simulink model "Free_Flight_ARDrone_joystick"  (R2016b)
settings: configuration reference "AR_Drone_ConfigSet" (kept outside this file)
undefined symbols (not defined in the file): DiscIntNeverNeededParam
libraries: dspnetwork x4, simulink x4, instrumentlib x2, AR_Drone_Actuators x2, AR_Drone_Sensors x1, AR_Drone_Positioning x1, etargetslib x1
settings Model: DataDictionary=ArDroneDataDictionary.sldd  SimulationMode=external  ExtModeTrigDuration=48000  Creator=nraman  LastModifiedBy=Miguel
settings ConfigSetRef: DDName=ArDroneDataDictionary.sldd

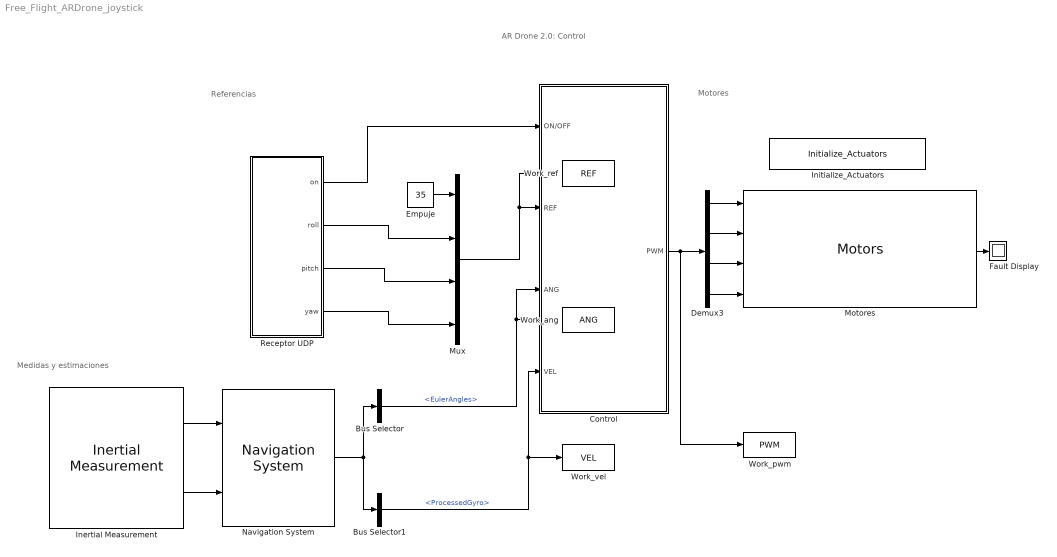
== system Free_Flight_ARDrone_joystick ==
  note: AR Drone 2.0: Control
  note: Motores
  note: Medidas y estimaciones
  note: Referencias
  Bus Selector : BusSelector  OutputSignals=EulerAngles
  Bus Selector1 : BusSelector  OutputSignals=ProcessedGyro
  Control : Subsystem
  Demux3 : Demux
  Empuje : Constant  Value=35
  Fault Display : Display
  Inertial Measurement : AR_Drone_Sensors/Inertial Measurement  Ts=1/400
  Initialize_Actuators : AR_Drone_Actuators/Initialize_Actuators  ShowSpec=on
  Motores : AR_Drone_Actuators/Motors
  Mux : Mux
  Navigation System : AR_Drone_Positioning/Navigation System
  Receptor UDP : Subsystem
  Work_ang : ToWorkspace  VariableName=ANG  SaveFormat=Structure With Time  SampleTime=0.0025
  Work_pwm : ToWorkspace  VariableName=PWM  SaveFormat=Structure With Time  SampleTime=0.0025
  Work_ref : ToWorkspace  VariableName=REF  SaveFormat=Structure With Time  SampleTime=0.0025
  Work_vel : ToWorkspace  VariableName=VEL  SaveFormat=Structure With Time  SampleTime=0.0025
  wires:
  Motores/1 -> Fault Display/1
  Demux3/1 -> Motores/1
  Demux3/2 -> Motores/2
  Demux3/3 -> Motores/3
  Demux3/4 -> Motores/4
  Inertial Measurement/1 -> Navigation System/1
  Inertial Measurement/2 -> Navigation System/2
  Navigation System/1 -> Bus Selector1/1, Bus Selector/1
  Bus Selector/1 -> Work_ang/1, Control/3(ANG)  "<EulerAngles>"
  Control/1(PWM) -> Work_pwm/1, Demux3/1
  Receptor UDP/1(on) -> Control/1(ON/OFF)
  Empuje/1 -> Mux/1
  Bus Selector1/1 -> Work_vel/1, Control/4(VEL)  "<ProcessedGyro>"
  Mux/1 -> Work_ref/1, Control/2(REF)
  Receptor UDP/2(roll) -> Mux/2
  Receptor UDP/3(pitch) -> Mux/3
  Receptor UDP/4(yaw) -> Mux/4

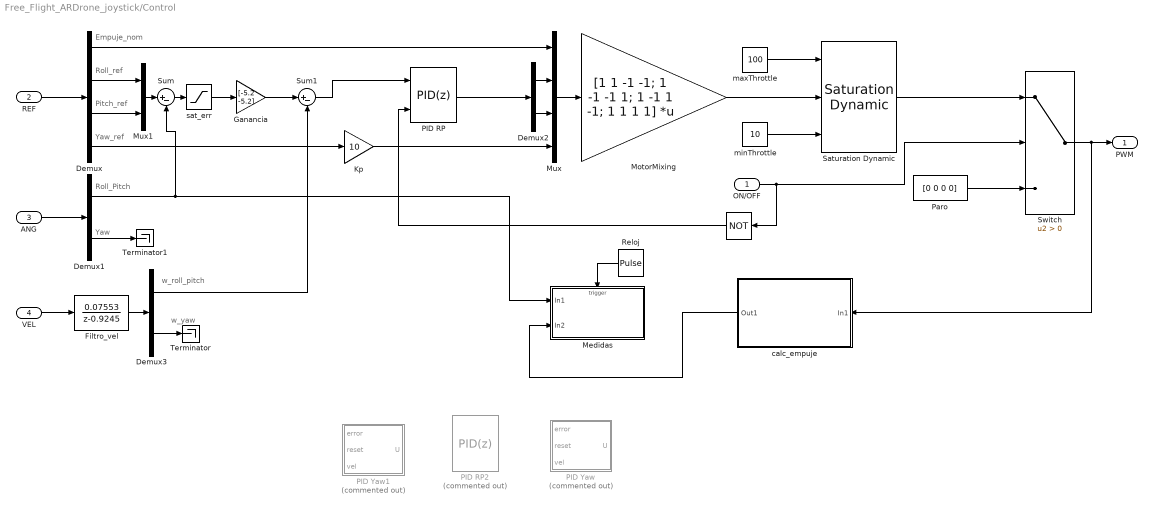
== system Free_Flight_ARDrone_joystick/Control ==
  note: Empuje_nom
  note: Roll_ref
  note: Pitch_ref
  note: Yaw_ref
  note: Roll_Pitch
  note: Yaw
  note: w_roll_pitch
  note: w_yaw
  ON/OFF : Inport
  REF : Inport  Port=2
  ANG : Inport  Port=3
  VEL : Inport  Port=4
  " " : Logic  Operator=NOT  AllPortsSameDT=off  OutDataTypeStr=boolean
  Demux : Demux
  Demux1 : Demux  Outputs=[2 1]
  Demux2 : Demux  Outputs=2
  Demux3 : Demux  Outputs=[2 1]
  Filtro_vel : DiscreteTransferFcn  Numerator=[0.07553]  Denominator=[1 -0.9245]
  Ganancia : Gain  Gain=[-5.2 -5.2]
  Kp : Gain  Gain=10
  Medidas : Subsystem
  MotorMixing : Gain  Gain=[1 1 -1 -1; 1 -1 -1 1; 1 -1 1 -1; 1 1 1 1]  Multiplication=Matrix(K*u)  ParamDataTypeStr=int16  OutDataTypeStr=int16
  Mux : Mux
  Mux1 : Mux  Inputs=2
  PID RP : simulink/Continuous/PID Controller  Controller=PID  TimeDomain=Discrete-time  SampleTime=-1  IntegratorMethod=Forward Euler  FilterMethod=Forward Euler  Form=Parallel  UseFilter=on  ControllerParametersSource=internal  P=0.5  I=0.3  D=-0.04  N=5  InitialConditionSource=internal  InitialConditionForIntegrator=0  InitialConditionForFilter=0  ExternalReset=level  LimitOutput=on  UpperSaturationLimit=30  LowerSaturationLimit=-30  LinearizeAsGain=on  AntiWindupMode=clamping  Kb=1  TrackingMode=off  Kt=1  PParamMin=[]  PParamMax=[]  IParamMin=[]  IParamMax=[]  DParamMin=[]  DParamMax=[]  NParamMin=[]  NParamMax=[]  KbParamMin=[]  KbParamMax=[]  KtParamMin=[]  KtParamMax=[]  POutMin=[]  POutMax=[]  IOutMin=[]  IOutMax=[]  DOutMin=[]  DOutMax=[]  NOutMin=[]  NOutMax=[]  KbOutMin=[]  KbOutMax=[]  KtOutMin=[]  KtOutMax=[]  IntegratorOutMin=[]  IntegratorOutMax=[]  FilterOutMin=[]  FilterOutMax=[]  SumOutMin=[]  SumOutMax=[]  SumI1OutMin=[]  SumI1OutMax=[]  SumI2OutMin=[]  SumI2OutMax=[]  SumI3OutMin=[]  SumI3OutMax=[]  SumDOutMin=[]  SumDOutMax=[]  SaturationOutMin=[]  SaturationOutMax=[]  IntegratorContinuousStateAttributes=''  IntegratorStateMustResolveToSignalObject=off  IntegratorRTWStateStorageClass=Auto  FilterContinuousStateAttributes=''  FilterStateMustResolveToSignalObject=off  FilterRTWStateStorageClass=Auto  DifferentiatorICPrevScaledInput=0  DifferentiatorOutMin=[]  DifferentiatorOutMax=[]
  PID RP2 : simulink/Continuous/PID Controller  Commented=on  Controller=PID  TimeDomain=Discrete-time  SampleTime=-1  IntegratorMethod=Forward Euler  FilterMethod=Forward Euler  Form=Parallel  UseFilter=on  ControllerParametersSource=internal  P=0.4  I=0.25  D=-0.05  N=5  InitialConditionSource=internal  InitialConditionForIntegrator=0  InitialConditionForFilter=0  ExternalReset=level  LimitOutput=on  UpperSaturationLimit=30  LowerSaturationLimit=-30  LinearizeAsGain=on  AntiWindupMode=clamping  Kb=1  TrackingMode=off  Kt=1  PParamMin=[]  PParamMax=[]  IParamMin=[]  IParamMax=[]  DParamMin=[]  DParamMax=[]  NParamMin=[]  NParamMax=[]  KbParamMin=[]  KbParamMax=[]  KtParamMin=[]  KtParamMax=[]  POutMin=[]  POutMax=[]  IOutMin=[]  IOutMax=[]  DOutMin=[]  DOutMax=[]  NOutMin=[]  NOutMax=[]  KbOutMin=[]  KbOutMax=[]  KtOutMin=[]  KtOutMax=[]  IntegratorOutMin=[]  IntegratorOutMax=[]  FilterOutMin=[]  FilterOutMax=[]  SumOutMin=[]  SumOutMax=[]  SumI1OutMin=[]  SumI1OutMax=[]  SumI2OutMin=[]  SumI2OutMax=[]  SumI3OutMin=[]  SumI3OutMax=[]  SumDOutMin=[]  SumDOutMax=[]  SaturationOutMin=[]  SaturationOutMax=[]  IntegratorContinuousStateAttributes=''  IntegratorStateMustResolveToSignalObject=off  IntegratorRTWStateStorageClass=Auto  FilterContinuousStateAttributes=''  FilterStateMustResolveToSignalObject=off  FilterRTWStateStorageClass=Auto  DifferentiatorICPrevScaledInput=0  DifferentiatorOutMin=[]  DifferentiatorOutMax=[]
  PID Yaw : Subsystem  Commented=on
  PID Yaw1 : Subsystem  Commented=on
  Paro : Constant  Value=[0 0 0 0]  OutDataTypeStr=int16
  Reloj : DiscretePulseGenerator  PulseType=Time based  Period=0.1  PulseWidth=50
  Saturation Dynamic : simulink/Discontinuities/Saturation Dynamic  OutMin=[]  OutMax=[]  OutDataTypeStr=Inherit: Same as second input  OutDataType=fixdt(1, 16)  OutScaling=2^-10  DoSatur=off
  Sum : Sum  Inputs=|+-
  Sum1 : Sum  Inputs=|+-
  Switch : Switch  Criteria=u2 > Threshold
  Terminator : Terminator
  Terminator1 : Terminator
  calc_empuje : Subsystem
  maxThrottle : Constant  Value=100  OutDataTypeStr=int16  SampleTime=-1
  minThrottle : Constant  Value=10  OutDataTypeStr=int16
  sat_err : Saturate  UpperLimit=[20 20]  LowerLimit=[-20 -20]
  PWM : Outport
  wires:
  MotorMixing/1 -> Saturation Dynamic/2
  Paro/1 -> Switch/3
  ON/OFF/1 -> " "/1, Switch/2
  Saturation Dynamic/1 -> Switch/1
  Mux/1 -> MotorMixing/1
  Switch/1 -> calc_empuje/1(In1), PWM/1
  minThrottle/1 -> Saturation Dynamic/3
  maxThrottle/1 -> Saturation Dynamic/1
  Demux/1 -> Mux/1
  ANG/1 -> Demux1/1
  VEL/1 -> Filtro_vel/1
  Kp/1 -> Mux/4
  Demux/2 -> Mux1/1
  Demux/3 -> Mux1/2
  Mux1/1 -> Sum/1
  Demux1/1 -> Sum/2, Medidas/1(In1)
  Demux/4 -> Kp/1
  sat_err/1 -> Ganancia/1
  Demux2/1 -> Mux/2
  Demux2/2 -> Mux/3
  Ganancia/1 -> Sum1/1
  Sum1/1 -> PID RP/1
  Sum/1 -> sat_err/1
  " "/1 -> PID RP/2
  PID RP/1 -> Demux2/1
  Demux3/1 -> Sum1/2
  Reloj/1 -> Medidas/Trigger
  calc_empuje/1(Out1) -> Medidas/2(In2)
  Filtro_vel/1 -> Demux3/1
  REF/1 -> Demux/1
  Demux3/2 -> Terminator/1
  Demux1/2 -> Terminator1/1

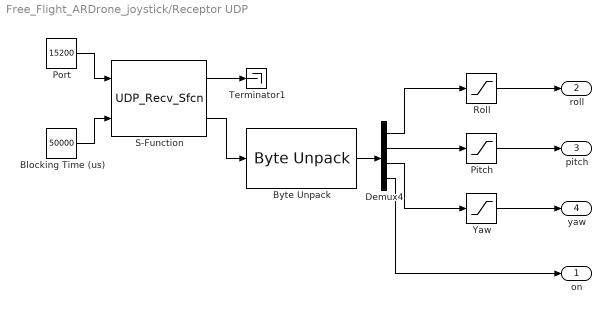
== system Free_Flight_ARDrone_joystick/Receptor UDP ==
  Blocking Time (us) : Constant  Value=50000  OutDataTypeStr=double
  Byte Unpack : etargetslib/Byte Unpack  dimensions={[4]}  datatypes={'double'}  byteAlign=1
  Demux4 : Demux
  Pitch : Saturate  UpperLimit=20  LowerLimit=-20
  Port : Constant  Value=15200  OutDataTypeStr=int32
  Roll : Saturate  UpperLimit=20  LowerLimit=-20
  S-Function : S-Function  FunctionName=UDP_Recv_Sfcn  Parameters=0.1  SFunctionDeploymentMode=off  EnableBusSupport=off
  Terminator1 : Terminator
  Yaw : Saturate  UpperLimit=1  LowerLimit=-1
  on : Outport
  roll : Outport  Port=2
  pitch : Outport  Port=3
  yaw : Outport  Port=4
  wires:
  Blocking Time (us)/1 -> S-Function/2
  S-Function/2 -> Byte Unpack/1
  Demux4/2 -> Pitch/1
  Demux4/1 -> Roll/1
  Demux4/4 -> on/1
  S-Function/1 -> Terminator1/1
  Byte Unpack/1 -> Demux4/1
  Demux4/3 -> Yaw/1
  Port/1 -> S-Function/1
  Roll/1 -> roll/1
  Pitch/1 -> pitch/1
  Yaw/1 -> yaw/1

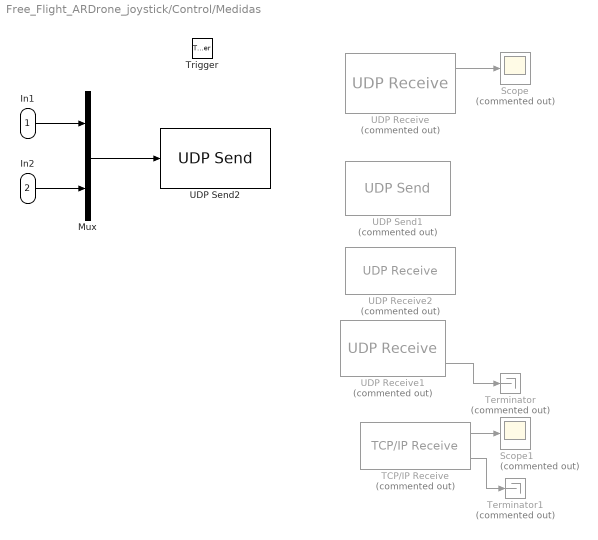
== system Free_Flight_ARDrone_joystick/Control/Medidas ==
  In1 : Inport
  In2 : Inport  Port=2
  Trigger : TriggerPort  VariantControl=Variant  PortDimensions=1
  Mux : Mux  Inputs=2
  Scope : Scope  Commented=on
  Scope1 : Scope  Commented=on
  TCP/IP Receive : instrumentlib/TCP//IP Receive  Commented=on  Host=192.168.1.2  Port=23  DataSize=[1 1]  EnableBlockingMode=off  Timeout=10  SampleTime=-1  DataType=double  ByteOrder=BigEndian
  Terminator : Terminator  Commented=on
  Terminator1 : Terminator  Commented=on
  UDP Receive : dspnetwork/UDP Receive  Commented=on  localURL='0.0.0.0'  localPort=51600  remoteURL='0.0.0.0'  remotePort=-1  recvBufferSize=32  dims=8  signalDatatype=uint8  isVarSize=off  showBlockingTime=on  blockingTime=0.1  sampletime=-1  blockPlatform=HOST
  UDP Receive1 : dspnetwork/UDP Receive  Priority=2  Commented=on  localURL='0.0.0.0'  localPort=50001  remoteURL='192.168.1.2'  remotePort=-1  recvBufferSize=16  dims=2  signalDatatype=double  isVarSize=off  showBlockingTime=off  blockingTime=0  sampletime=-1
  UDP Receive2 : instrumentlib/UDP Receive  Priority=2  Commented=on  Host=127.0.0.1  Port=36864  LocalPort=36880  DataSize=8  EnableBlockingMode=off  Timeout=10  SampleTime=-1  DataType=double  ByteOrder=LittleEndian
  UDP Send1 : dspnetwork/UDP Send  Commented=on  remoteURL='192.168.1.2'  remotePort=50000  localURL='0.0.0.0'  localPortSource=Automatically determine  localPort=2048  sampletime=-1  separateLengthPort=0
  UDP Send2 : dspnetwork/UDP Send  remoteURL='192.168.1.2'  remotePort=50000  localURL='0.0.0.0'  localPortSource=Automatically determine  localPort=-1  sampletime=-1  blockPlatform=HOST  separateLengthPort=0
  wires:
  TCP/IP Receive/1 -> Scope1/1
  TCP/IP Receive/2 -> Terminator1/1
  UDP Receive1/2 -> Terminator/1
  UDP Receive/1 -> Scope/1
  In1/1 -> Mux/1
  In2/1 -> Mux/2
  Mux/1 -> UDP Send2/1

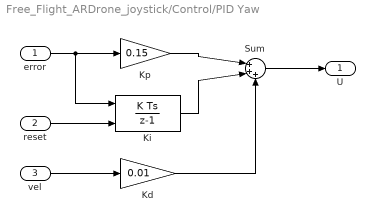
== system Free_Flight_ARDrone_joystick/Control/PID Yaw ==
  error : Inport
  reset : Inport  Port=2
  vel : Inport  Port=3
  Kd : Gain  Gain=0.01
  Ki : DiscreteIntegrator  gainval=0.1  ExternalReset=level  InitialConditionSetting=State (most efficient)  SampleTime=-1  LimitOutput=on  UpperSaturationLimit=10  LowerSaturationLimit=-10  ICPrevOutput=DiscIntNeverNeededParam  ICPrevScaledInput=DiscIntNeverNeededParam
  Kp : Gain  Gain=0.15
  Sum : Sum  Inputs=|+++
  U : Outport
  wires:
  error/1 -> Ki/1, Kp/1
  Ki/1 -> Sum/2
  reset/1 -> Ki/2
  vel/1 -> Kd/1
  Kd/1 -> Sum/3
  Kp/1 -> Sum/1
  Sum/1 -> U/1

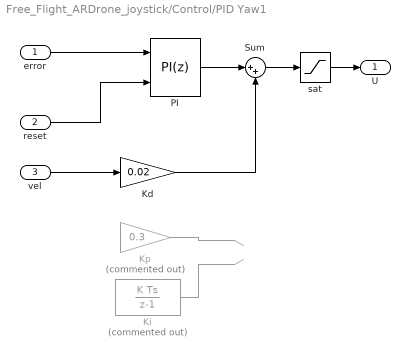
== system Free_Flight_ARDrone_joystick/Control/PID Yaw1 ==
  error : Inport
  reset : Inport  Port=2
  vel : Inport  Port=3
  Kd : Gain  Gain=0.02
  Ki : DiscreteIntegrator  Commented=on  gainval=0.3  ExternalReset=level  InitialConditionSetting=State (most efficient)  SampleTime=-1  LimitOutput=on  UpperSaturationLimit=10  LowerSaturationLimit=-10  ICPrevOutput=DiscIntNeverNeededParam  ICPrevScaledInput=DiscIntNeverNeededParam
  Kp : Gain  Commented=on  Gain=0.3
  PI : simulink/Continuous/PID Controller  Controller=PI  TimeDomain=Discrete-time  SampleTime=-1  IntegratorMethod=Forward Euler  FilterMethod=Forward Euler  Form=Parallel  UseFilter=on  ControllerParametersSource=internal  P=0.3  I=0.3  D=-0.05  N=5  InitialConditionSource=internal  InitialConditionForIntegrator=0  InitialConditionForFilter=0  ExternalReset=level  LimitOutput=on  UpperSaturationLimit=20  LowerSaturationLimit=-20  LinearizeAsGain=on  AntiWindupMode=clamping  Kb=1  TrackingMode=off  Kt=1  PParamMin=[]  PParamMax=[]  IParamMin=[]  IParamMax=[]  DParamMin=[]  DParamMax=[]  NParamMin=[]  NParamMax=[]  KbParamMin=[]  KbParamMax=[]  KtParamMin=[]  KtParamMax=[]  POutMin=[]  POutMax=[]  IOutMin=[]  IOutMax=[]  DOutMin=[]  DOutMax=[]  NOutMin=[]  NOutMax=[]  KbOutMin=[]  KbOutMax=[]  KtOutMin=[]  KtOutMax=[]  IntegratorOutMin=[]  IntegratorOutMax=[]  FilterOutMin=[]  FilterOutMax=[]  SumOutMin=[]  SumOutMax=[]  SumI1OutMin=[]  SumI1OutMax=[]  SumI2OutMin=[]  SumI2OutMax=[]  SumI3OutMin=[]  SumI3OutMax=[]  SumDOutMin=[]  SumDOutMax=[]  SaturationOutMin=[]  SaturationOutMax=[]  IntegratorContinuousStateAttributes=''  IntegratorStateMustResolveToSignalObject=off  IntegratorRTWStateStorageClass=Auto  FilterContinuousStateAttributes=''  FilterStateMustResolveToSignalObject=off  FilterRTWStateStorageClass=Auto  DifferentiatorICPrevScaledInput=0  DifferentiatorOutMin=[]  DifferentiatorOutMax=[]
  Sum : Sum  Inputs=|++
  sat : Saturate  UpperLimit=20  LowerLimit=-20
  U : Outport
  wires:
  error/1 -> PI/1
  reset/1 -> PI/2
  vel/1 -> Kd/1
  Kd/1 -> Sum/2
  Sum/1 -> sat/1
  sat/1 -> U/1
  Ki/1 -> ?
  Kp/1 -> ?
  PI/1 -> Sum/1

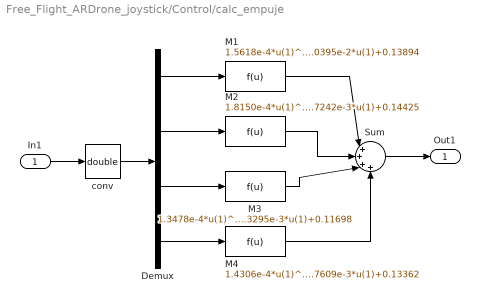
== system Free_Flight_ARDrone_joystick/Control/calc_empuje ==
  In1 : Inport
  Demux : Demux
  M1 : Fcn  Expr=1.5618e-4*u(1)^2+1.0395e-2*u(1)+0.13894
  M2 : Fcn  Expr=1.8150e-4*u(1)^2+8.7242e-3*u(1)+0.14425
  M3 : Fcn  Expr=1.3478e-4*u(1)^2+7.3295e-3*u(1)+0.11698
  M4 : Fcn  Expr=1.4306e-4*u(1)^2+5.7609e-3*u(1)+0.13362
  Sum : Sum  Inputs=|++++
  conv : DataTypeConversion  OutDataTypeStr=double  RndMeth=Nearest
  Out1 : Outport
  wires:
  Demux/1 -> M1/1
  Demux/2 -> M2/1
  Demux/3 -> M3/1
  Demux/4 -> M4/1
  M1/1 -> Sum/1
  M2/1 -> Sum/2
  M3/1 -> Sum/3
  M4/1 -> Sum/4
  Sum/1 -> Out1/1
  conv/1 -> Demux/1
  In1/1 -> conv/1
